simulink subsystem "Actuator_RW"  (R2025a)
settings: Solver=VariableStepAuto  StartTime=0.0  StopTime=10.0  RelTol=1e-3
undefined symbols (not defined in the file): J_wheel, Omega_wheel_max, tau_wheel_max
settings Model: Creator=Jackt  LastModifiedBy=Jackt

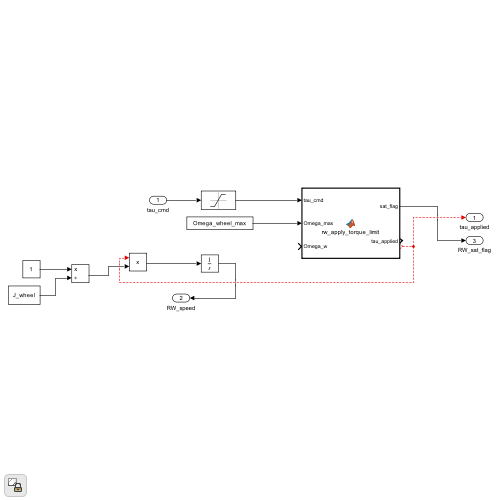
[thumbnail: Simulink's stored preview of the top-level diagram]
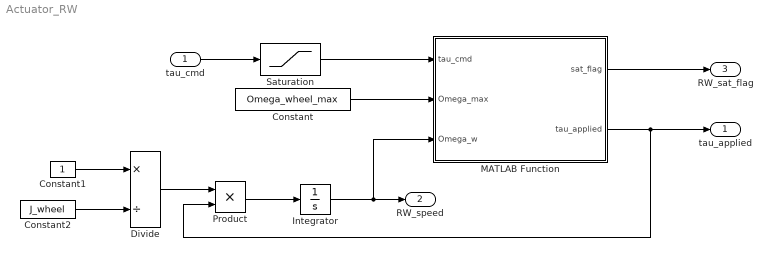
== system Actuator_RW ==
  tau_cmd : Inport
  Constant : Constant  Value=Omega_wheel_max
  Constant1 : Constant
  Constant2 : Constant  Value=J_wheel  VectorParams1D=off
  Divide : Product  Inputs=*/
  Integrator : Integrator
  MATLAB Function : MATLAB Function  TreatAsAtomicUnit=on
  Product : Product
  Saturation : Saturate  UpperLimit=tau_wheel_max  LowerLimit=-tau_wheel_max
  tau_applied : Outport
  RW_speed : Outport  Port=2
  RW_sat_flag : Outport  Port=3
  wires:
  Saturation/1 -> MATLAB Function/1(tau_cmd)
  tau_cmd/1 -> Saturation/1
  Product/1 -> Integrator/1
  Integrator/1 -> MATLAB Function/3(Omega_w), RW_speed/1
  Divide/1 -> Product/1
  Constant1/1 -> Divide/1
  Constant2/1 -> Divide/2
  MATLAB Function/2(tau_applied) -> tau_applied/1, Product/2
  MATLAB Function/1(sat_flag) -> RW_sat_flag/1
  Constant/1 -> MATLAB Function/2(Omega_max)

== matlab function Actuator_RW/MATLAB Function ==
  data: sat_flag output; tau_cmd input; tau_applied output; Omega_max input; Omega_w input
function [sat_flag, tau_applied]   = rw_apply_torque_limit(tau_cmd, Omega_max, Omega_w)
%RW_APPLY_TORQUE_LIMIT

%Force shapes
tau_cmd  = reshape(tau_cmd,  [3 1]);
Omega_w  = reshape(Omega_w,  [3 1]);

%Preallocate output
tau_applied = zeros(3,1);
sat_flag = zeros(3, 1);

%Small tolerance to avoid chattering at the limit
tol = 1e-6;

%Axis-by-axis limiting
for i = 1:3
    tau_i = tau_cmd(i);
    omega_i = Omega_w(i);

    %If wheel is at/over +Omega_max AND commanded torque would increase speed -> block
    if (omega_i >= (Omega_max - tol) && tau_i > 0)
        tau_applied(i) = 0;
        sat_flag(i) = 1;

    %If wheel is at/over -Omega_max AND commanded torque would decrease speed further -> block
    elseif (omega_i <= (-Omega_max + tol) && tau_i < 0)
        tau_applied(i) = 0;
        sat_flag(i) = 1;

    %Otherwise allow commanded torque
    else
        tau_applied(i) = tau_i;
    end
end

end
